simulink model "steercont_SAVIK_2019b_"  (R2020a)
settings: Solver=FixedStepAuto  StartTime=0.0  StopTime=270  FixedStep=stept  RelTol=1e-3
model workspace (MAT data in the model file):
  ip = Simulink.Signal
  ip.DataType = 'double'
  ip.Dimensions = [1 2]
  ip.DimensionsMode = 'auto'
  ip.Complexity = 'real'
  ip.SampleTime = -1
  ip.SamplingMode = 'auto'
values from neighbouring files (symbols this model uses):
  IC_theta0 = gamma_1+IC_theta1    (= 4.71238898038)    [purepursuit_waypoints.m]
  IC_theta1 = (3*pi)/2    (= 4.71238898038)    [purepursuit_waypoints.m]
  IC_x0 = IC_x0f-L_0f*cos(IC_theta0)    [purepursuit_waypoints.m]
  IC_x1 = 0    [purepursuit_waypoints.m]
  IC_y0 = IC_y0f-L_0f*sin(IC_theta0)    [purepursuit_waypoints.m]
  IC_y1 = 0    [purepursuit_waypoints.m]
  L_0b = 0.48    [purepursuit_waypoints.m]
  L_0f = 3.8    [purepursuit_waypoints.m]
  L_1f = 7.21    [purepursuit_waypoints.m]
  LD = 15    [purepursuit_waypoints.m]
  stept = 0.01    [purepursuit_waypoints.m]
  v_0 = -1    [purepursuit_waypoints.m]
  wayp = [0 0;0 20;20 20;20 -40; -40 -40; 0 -80]    [purepursuit_waypoints.m]
undefined symbols (not defined in the file or in its folder): DiscIntNeverNeededParam
settings Model: PauseTimes=0  OrderedModelArguments=off  Creator=giridhar  LastModifiedBy=giridhar
settings SolverCC: AlgebraicLoopSolver=LineSearch  MinimalZcImpactIntegration=on
settings DebuggingCC: ReadBeforeWriteMsg=DisableAll  WriteAfterWriteMsg=DisableAll  WriteAfterReadMsg=DisableAll  MultiTaskDSMMsg=none  SFUnusedDataAndEventsDiag=none
settings ModelReferenceCC: UpdateModelReferenceTargets=IfOutOfDate
settings SFSimCC: SFSimEcho=off

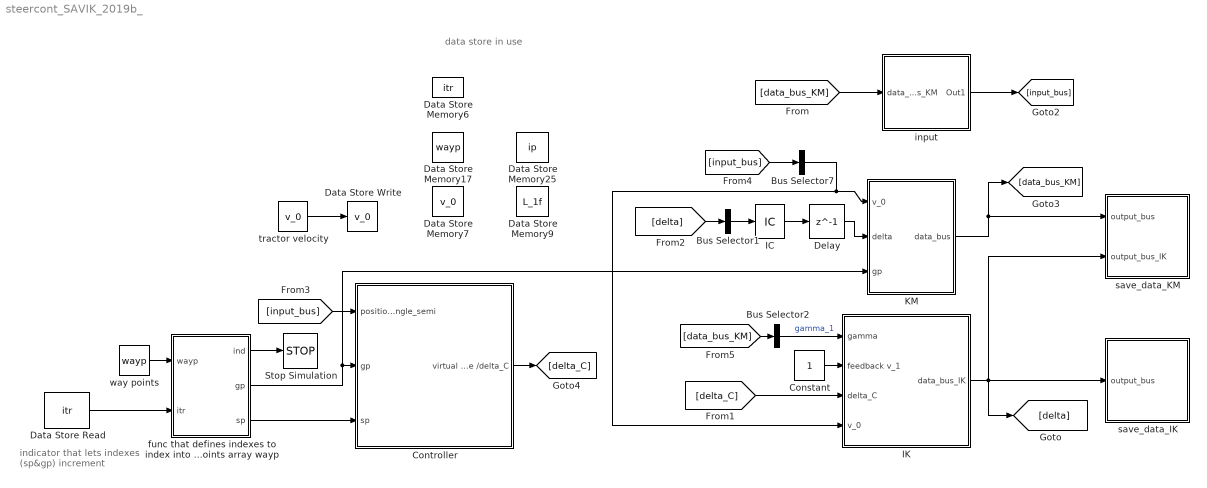
== system steercont_SAVIK_2019b_ ==
  note: indicator that lets indexes
      | (sp&gp) increment
  note: data store in use
  Bus Selector1 : BusSelector  OutputSignals=angle.steering_angle  OutputAsBus=on
  Bus Selector2 : BusSelector  OutputSignals=angle.articulation_angle  OutputAsBus=on
  Bus Selector7 : BusSelector  OutputSignals=u_0  OutputAsBus=on
  Constant : Constant
  Controller : Subsystem
  Data Store Memory17 : DataStoreMemory  DataStoreName=wayp  ReadBeforeWriteMsg=warning  WriteAfterWriteMsg=warning  WriteAfterReadMsg=warning  InitialValue=wayp  VectorParams1D=off  ShowAdditionalParam=off  OutDataTypeStr=double
  Data Store Memory25 : DataStoreMemory  DataStoreName=ip  ReadBeforeWriteMsg=warning  WriteAfterWriteMsg=warning  WriteAfterReadMsg=warning  InitialValue=[0 0]  VectorParams1D=off  ShowAdditionalParam=off  OutDataTypeStr=double  Dimensions=[1 2]  StateMustResolveToSignalObject=on
  Data Store Memory6 : DataStoreMemory  DataStoreName=itr  ReadBeforeWriteMsg=warning  WriteAfterWriteMsg=warning  WriteAfterReadMsg=warning  VectorParams1D=off  ShowAdditionalParam=off  OutDataTypeStr=double
  Data Store Memory7 : DataStoreMemory  DataStoreName=v_0  ReadBeforeWriteMsg=warning  WriteAfterWriteMsg=warning  WriteAfterReadMsg=warning  InitialValue=v_0  VectorParams1D=off  ShowAdditionalParam=off  OutDataTypeStr=double  Dimensions=[1 1]
  Data Store Memory9 : DataStoreMemory  DataStoreName=L_1f  ReadBeforeWriteMsg=warning  WriteAfterWriteMsg=warning  WriteAfterReadMsg=warning  InitialValue=7.21  VectorParams1D=off  ShowAdditionalParam=off  OutDataTypeStr=double  Dimensions=[1 1]
  Data Store Read : DataStoreRead  DataStoreName=itr
  Data Store Write : DataStoreWrite  DataStoreName=v_0
  Delay : Delay  DelayLength=1
  IC : InitialCondition  Value=0
  IK : Subsystem  SystemSampleTime=0.8
  KM : Subsystem  SystemSampleTime=0.8
  Stop Simulation : Stop
  func that defines indexes to index into waypoints array wayp : MATLAB Function
  input : Subsystem
  save_data_IK : Subsystem
  save_data_KM : Subsystem
  tractor velocity : Constant  Value=v_0
  way points : Constant  Value=wayp
  wires:
  [data_bus_KM] -> Bus Selector2/1
  input/1(Out1) -> [input_bus]
  KM/1(data_bus) -> [data_bus_KM], save_data_KM/1(output_bus)
  [delta] -> Bus Selector1/1
  IC/1 -> Delay/1
  Bus Selector2/1 -> IK/1(gamma)  "gamma_1"
  [input_bus] -> Controller/1(positions_yawangle_semi)
  Delay/1 -> KM/2(delta)
  Controller/1(virtual steer angle /delta_C) -> [delta_C]
  [input_bus] -> Bus Selector7/1
  [delta_C] -> IK/3(delta_C)
  [data_bus_KM] -> input/1(data_bus_KM)
  Bus Selector7/1 -> IK/4(v_0), KM/1(v_0)
  Bus Selector1/1 -> IC/1
  Constant/1 -> IK/2(feedback v_1)
  way points/1 -> func that defines indexes to index into waypoints array wayp/1(wayp)
  Data Store Read/1 -> func that defines indexes to index into waypoints array wayp/2(itr)
  func that defines indexes to index into waypoints array wayp/2(gp) -> Controller/2(gp), KM/3(gp)
  func that defines indexes to index into waypoints array wayp/3(sp) -> Controller/3(sp)
  func that defines indexes to index into waypoints array wayp/1(ind) -> Stop Simulation/1
  tractor velocity/1 -> Data Store Write/1
  IK/1(data_bus_IK) -> save_data_IK/1(output_bus), save_data_KM/2("output_bus_IK "), [delta]

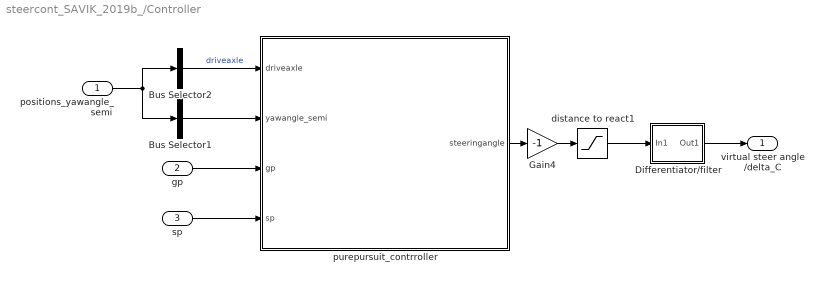
== system steercont_SAVIK_2019b_/Controller ==
  positions_yawangle_semi : Inport
  gp : Inport  Port=2
  sp : Inport  Port=3
  Bus Selector1 : BusSelector  OutputSignals=yawangle_semi  OutputAsBus=on
  Bus Selector2 : BusSelector  OutputSignals=positions  OutputAsBus=on
  Differentiator/filter : Subsystem  mask{ts=13.5}
      mask prompts: ts "response_time"
      mask init:
      | c=(3*pi/ts)^2;
  Gain4 : Gain  Gain=-1
  distance to react1 : Saturate  UpperLimit=1  LowerLimit=-1
  purepursuit_contrroller : Subsystem
  virtual steer angle /delta_C : Outport  PortDimensions=[1,1]  VectorParamsAs1DForOutWhenUnconnected=off
  wires:
  distance to react1/1 -> Differentiator/filter/1(In1)
  purepursuit_contrroller/1(steeringangle) -> Gain4/1
  Bus Selector2/1 -> purepursuit_contrroller/1(driveaxle)  "driveaxle"
  positions_yawangle_semi/1 -> Bus Selector1/1, Bus Selector2/1
  gp/1 -> purepursuit_contrroller/3(gp)
  sp/1 -> purepursuit_contrroller/4(sp)
  Gain4/1 -> distance to react1/1
  Bus Selector1/1 -> purepursuit_contrroller/2(yawangle_semi)
  Differentiator/filter/1(Out1) -> virtual steer angle /delta_C/1

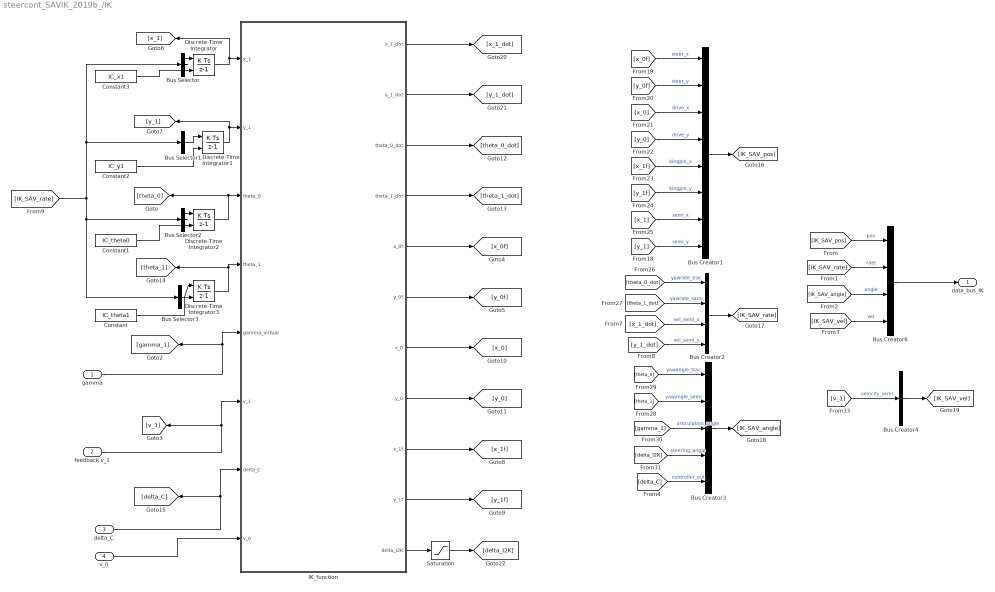
== system steercont_SAVIK_2019b_/IK ==
  gamma : Inport
  feedback v_1 : Inport  Port=2
  delta_C : Inport  Port=3
  v_0 : Inport  Port=4
  Bus Creator1 : BusCreator  Inputs=8
  Bus Creator2 : BusCreator  Inputs=4
  Bus Creator3 : BusCreator  Inputs=5
  Bus Creator4 : BusCreator  Inputs=1
  Bus Creator6 : BusCreator  Inputs=4
  Bus Selector : BusSelector  OutputSignals=vel_semi_x  OutputAsBus=on
  Bus Selector1 : BusSelector  OutputSignals=vel_semi_y  OutputAsBus=on
  Bus Selector2 : BusSelector  OutputSignals=yawrate_trac  OutputAsBus=on
  Bus Selector3 : BusSelector  OutputSignals=yawrate_semi  OutputAsBus=on
  Constant : Constant  Value=IC_theta1
  Constant1 : Constant  Value=IC_theta0
  Constant2 : Constant  Value=IC_y1
  Constant3 : Constant  Value=IC_x1
  Discrete-Time Integrator : DiscreteIntegrator  InitialConditionSource=external  InitialCondition=IC_x1  SampleTime=-1  ICPrevOutput=DiscIntNeverNeededParam  ICPrevScaledInput=DiscIntNeverNeededParam
  Discrete-Time Integrator1 : DiscreteIntegrator  InitialConditionSource=external  InitialCondition=IC_y1  SampleTime=-1  ICPrevOutput=DiscIntNeverNeededParam  ICPrevScaledInput=DiscIntNeverNeededParam
  Discrete-Time Integrator2 : DiscreteIntegrator  InitialConditionSource=external  InitialCondition=IC_theta0  SampleTime=-1  ICPrevOutput=DiscIntNeverNeededParam  ICPrevScaledInput=DiscIntNeverNeededParam
  Discrete-Time Integrator3 : DiscreteIntegrator  InitialConditionSource=external  InitialCondition=IC_theta1  SampleTime=-1  ICPrevOutput=DiscIntNeverNeededParam  ICPrevScaledInput=DiscIntNeverNeededParam
  IK_function : MATLAB Function  TreatAsAtomicUnit=on
  Saturation : Saturate  UpperLimit=0.7  LowerLimit=-0.7
  data_bus_IK : Outport  VectorParamsAs1DForOutWhenUnconnected=off
  wires:
  IK_function/7(x_0) -> [x_0]
  IK_function/8(y_0) -> [y_0]
  IK_function/1(x_1_dot) -> [x_1_dot]
  IK_function/10(y_1f) -> [y_1f]
  IK_function/9(x_1f) -> [x_1f]
  Discrete-Time Integrator/1 -> [x_1], IK_function/1(x_1)
  Discrete-Time Integrator1/1 -> [y_1], IK_function/2(y_1)
  gamma/1 -> [gamma_1], IK_function/5(gamma_virtual)
  IK_function/2(y_1_dot) -> [y_1_dot]
  delta_C/1 -> IK_function/7(delta_C), [delta_C]
  Discrete-Time Integrator3/1 -> IK_function/4(theta_1), [theta_1]
  IK_function/5(x_0f) -> [x_0f]
  IK_function/6(y_0f) -> [y_0f]
  [y_0f] -> Bus Creator1/2  "steer_y"
  [x_1f] -> Bus Creator1/5  "kingpin_x"
  Bus Creator6/1 -> data_bus_IK/1
  [v_1] -> Bus Creator4/1  "velocity_semi"
  [x_0] -> Bus Creator1/3  "drive_x"
  [y_1f] -> Bus Creator1/6  "kingpin_y"
  [x_0f] -> Bus Creator1/1  "steer_x"
  [y_0] -> Bus Creator1/4  "drive_y"
  Bus Creator3/1 -> [IK_SAV_angle]
  [theta_0_dot] -> Bus Creator2/1  "yawrate_trac"
  [theta_1_dot] -> Bus Creator2/2  "yawrate_semi"
  Discrete-Time Integrator2/1 -> [theta_0], IK_function/3(theta_0)
  [IK_SAV_rate] -> Bus Selector/1, Bus Selector1/1, Bus Selector3/1, Bus Selector2/1
  Bus Creator2/1 -> [IK_SAV_rate]
  Bus Creator1/1 -> [IK_SAV_pos]
  [delta_I2K] -> Bus Creator3/4  "steering_angle"
  [gamma_1] -> Bus Creator3/3  "articulation_angle"
  Bus Creator4/1 -> [IK_SAV_vel]
  [theta_1] -> Bus Creator3/2  "yawangle_semi"
  [IK_SAV_rate] -> Bus Creator6/2  "rate"
  [theta_0] -> Bus Creator3/1  "yawangle_trac"
  [IK_SAV_pos] -> Bus Creator6/1  "pos"
  [IK_SAV_angle] -> Bus Creator6/3  "angle"
  [IK_SAV_vel] -> Bus Creator6/4  "vel"
  Bus Selector3/1 -> Discrete-Time Integrator3/1
  Bus Selector2/1 -> Discrete-Time Integrator2/1
  Bus Selector/1 -> Discrete-Time Integrator/1
  Bus Selector1/1 -> Discrete-Time Integrator1/1
  [y_1_dot] -> Bus Creator2/4  "vel_semi_y"
  [x_1_dot] -> Bus Creator2/3  "vel_semi_x"
  IK_function/11(delta_I2K) -> Saturation/1
  [delta_C] -> Bus Creator3/5  "controller_out"
  feedback v_1/1 -> [v_1], IK_function/6(v_1)
  Saturation/1 -> [delta_I2K]
  [y_1] -> Bus Creator1/8  "semi_y"
  [x_1] -> Bus Creator1/7  "semi_x"
  Constant/1 -> Discrete-Time Integrator3/2
  Constant1/1 -> Discrete-Time Integrator2/2
  Constant2/1 -> Discrete-Time Integrator1/2
  Constant3/1 -> Discrete-Time Integrator/2
  v_0/1 -> IK_function/8(v_0)
  IK_function/4(theta_1_dot) -> [theta_1_dot]
  IK_function/3(theta_0_dot) -> [theta_0_dot]

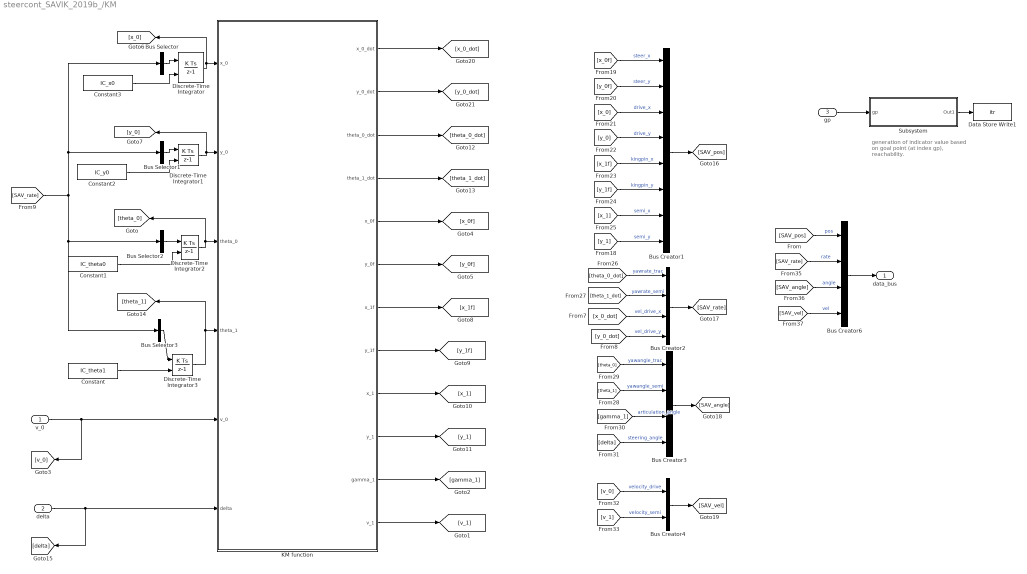
== system steercont_SAVIK_2019b_/KM ==
  note: generation of indicator value
      | based on goal point (at index gp),
      | reachability.
  v_0 : Inport
  delta : Inport  Port=2
  gp : Inport  Port=3
  Bus Creator1 : BusCreator  Inputs=8
  Bus Creator2 : BusCreator  Inputs=4
  Bus Creator3 : BusCreator  Inputs=4
  Bus Creator4 : BusCreator  Inputs=2
  Bus Creator6 : BusCreator  Inputs=4
  Bus Selector : BusSelector  OutputSignals=vel_drive_x  OutputAsBus=on
  Bus Selector1 : BusSelector  OutputSignals=vel_drive_y  OutputAsBus=on
  Bus Selector2 : BusSelector  OutputSignals=yawrate_trac  OutputAsBus=on
  Bus Selector3 : BusSelector  OutputSignals=yawrate_semi  OutputAsBus=on
  Constant : Constant  Value=IC_theta1
  Constant1 : Constant  Value=IC_theta0
  Constant2 : Constant  Value=IC_y0
  Constant3 : Constant  Value=IC_x0
  Data Store Write1 : DataStoreWrite  DataStoreName=itr
  Discrete-Time Integrator : DiscreteIntegrator  InitialConditionSource=external  InitialCondition=IC_x0  SampleTime=-1  ICPrevOutput=DiscIntNeverNeededParam  ICPrevScaledInput=DiscIntNeverNeededParam
  Discrete-Time Integrator1 : DiscreteIntegrator  InitialConditionSource=external  InitialCondition=IC_y0  SampleTime=-1  ICPrevOutput=DiscIntNeverNeededParam  ICPrevScaledInput=DiscIntNeverNeededParam
  Discrete-Time Integrator2 : DiscreteIntegrator  InitialConditionSource=external  InitialCondition=IC_theta0  SampleTime=-1  ICPrevOutput=DiscIntNeverNeededParam  ICPrevScaledInput=DiscIntNeverNeededParam
  Discrete-Time Integrator3 : DiscreteIntegrator  InitialConditionSource=external  InitialCondition=IC_theta1  SampleTime=-1  ICPrevOutput=DiscIntNeverNeededParam  ICPrevScaledInput=DiscIntNeverNeededParam
  KM function : MATLAB Function  TreatAsAtomicUnit=on
  Subsystem : Subsystem
  data_bus : Outport  VectorParamsAs1DForOutWhenUnconnected=off
  wires:
  KM function/9(x_1) -> [x_1]
  KM function/10(y_1) -> [y_1]
  KM function/1(x_0_dot) -> [x_0_dot]
  KM function/8(y_1f) -> [y_1f]
  KM function/7(x_1f) -> [x_1f]
  Discrete-Time Integrator/1 -> KM function/1(x_0), [x_0]
  Discrete-Time Integrator1/1 -> KM function/2(y_0), [y_0]
  KM function/11(gamma_1) -> [gamma_1]
  KM function/2(y_0_dot) -> [y_0_dot]
  delta/1 -> [delta], KM function/6(delta)
  Discrete-Time Integrator3/1 -> [theta_1], KM function/4(theta_1)
  KM function/5(x_0f) -> [x_0f]
  KM function/6(y_0f) -> [y_0f]
  v_0/1 -> [v_0], KM function/5(v_0)
  [y_0f] -> Bus Creator1/2  "steer_y"
  [x_1f] -> Bus Creator1/5  "kingpin_x"
  Bus Creator6/1 -> data_bus/1
  [v_1] -> Bus Creator4/2  "velocity_semi"
  [x_0] -> Bus Creator1/3  "drive_x"
  [y_1f] -> Bus Creator1/6  "kingpin_y"
  [x_0f] -> Bus Creator1/1  "steer_x"
  [y_0] -> Bus Creator1/4  "drive_y"
  Bus Creator3/1 -> [SAV_angle]
  [v_0] -> Bus Creator4/1  "velocity_drive"
  [theta_0_dot] -> Bus Creator2/1  "yawrate_trac"
  [theta_1_dot] -> Bus Creator2/2  "yawrate_semi"
  Discrete-Time Integrator2/1 -> [theta_0], KM function/3(theta_0)
  [SAV_rate] -> Bus Selector/1, Bus Selector1/1, Bus Selector3/1, Bus Selector2/1
  Bus Creator2/1 -> [SAV_rate]
  Bus Creator1/1 -> [SAV_pos]
  [delta] -> Bus Creator3/4  "steering_angle"
  [gamma_1] -> Bus Creator3/3  "articulation_angle"
  Bus Creator4/1 -> [SAV_vel]
  [theta_1] -> Bus Creator3/2  "yawangle_semi"
  [SAV_rate] -> Bus Creator6/2  "rate"
  [theta_0] -> Bus Creator3/1  "yawangle_trac"
  [SAV_pos] -> Bus Creator6/1  "pos"
  [SAV_angle] -> Bus Creator6/3  "angle"
  [SAV_vel] -> Bus Creator6/4  "vel"
  Bus Selector3/1 -> Discrete-Time Integrator3/1
  Bus Selector2/1 -> Discrete-Time Integrator2/1
  Bus Selector/1 -> Discrete-Time Integrator/1
  Bus Selector1/1 -> Discrete-Time Integrator1/1
  [y_0_dot] -> Bus Creator2/4  "vel_drive_y"
  [x_0_dot] -> Bus Creator2/3  "vel_drive_x"
  KM function/12(v_1) -> [v_1]
  [x_1] -> Bus Creator1/7  "semi_x"
  [y_1] -> Bus Creator1/8  "semi_y"
  Constant3/1 -> Discrete-Time Integrator/2
  Constant/1 -> Discrete-Time Integrator3/2
  Constant2/1 -> Discrete-Time Integrator1/2
  Constant1/1 -> Discrete-Time Integrator2/2
  Subsystem/1(Out1) -> Data Store Write1/1
  gp/1 -> Subsystem/1(gp)
  KM function/3(theta_0_dot) -> [theta_0_dot]
  KM function/4(theta_1_dot) -> [theta_1_dot]

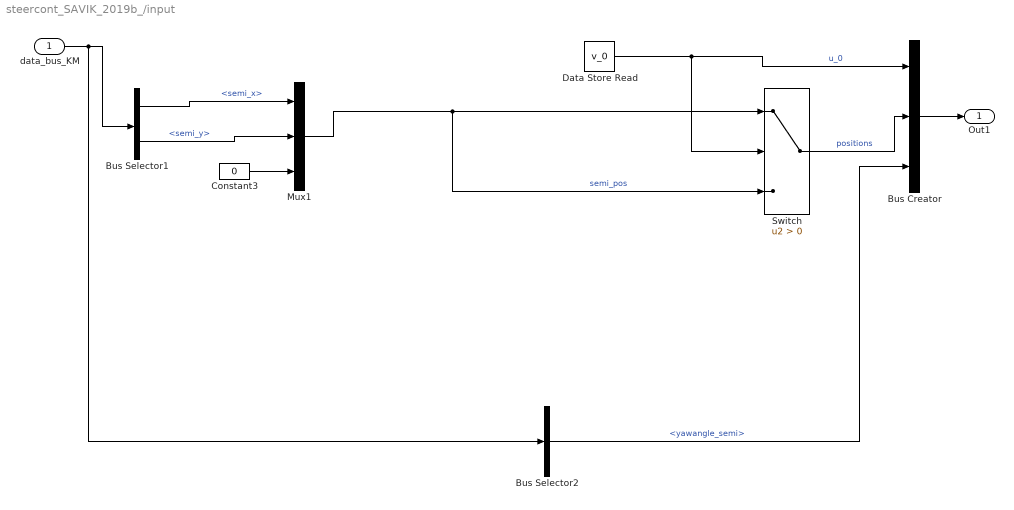
== system steercont_SAVIK_2019b_/input ==
  data_bus_KM : Inport
  Bus Creator : BusCreator  Inputs=3
  Bus Selector1 : BusSelector  OutputSignals=pos.semi_x,pos.semi_y
  Bus Selector2 : BusSelector  OutputSignals=angle.yawangle_semi
  Constant3 : Constant  Value=0
  Data Store Read : DataStoreRead  DataStoreName=v_0
  Mux1 : Mux  Inputs=3
  Switch : Switch  Criteria=u2 > Threshold
  Out1 : Outport  VectorParamsAs1DForOutWhenUnconnected=off
  wires:
  Data Store Read/1 -> Switch/2, Bus Creator/1  "u_0"
  Bus Creator/1 -> Out1/1
  Constant3/1 -> Mux1/3
  data_bus_KM/1 -> Bus Selector2/1, Bus Selector1/1
  Bus Selector1/1 -> Mux1/1  "<semi_x>"
  Bus Selector1/2 -> Mux1/2  "<semi_y>"
  Mux1/1 -> Switch/1, Switch/3  "semi_pos"
  Switch/1 -> Bus Creator/2  "positions"
  Bus Selector2/1 -> Bus Creator/3  "<yawangle_semi>"

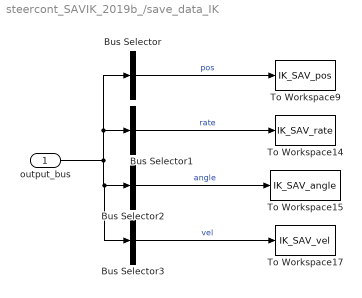
== system steercont_SAVIK_2019b_/save_data_IK ==
  output_bus : Inport
  Bus Selector : BusSelector  OutputSignals=pos.steer_x,pos.steer_y,pos.drive_x,pos.drive_y,pos.kingpin_x,pos.kingpin_y,pos.semi_x,pos.semi_y  OutputAsBus=on
  Bus Selector1 : BusSelector  OutputSignals=rate.yawrate_trac,rate.yawrate_semi,rate.vel_semi_x,rate.vel_semi_y  OutputAsBus=on
  Bus Selector2 : BusSelector  OutputSignals=angle.yawangle_trac,angle.yawangle_semi,angle.articulation_angle,angle.steering_angle,angle.controller_out  OutputAsBus=on
  Bus Selector3 : BusSelector  OutputSignals=vel.velocity_semi  OutputAsBus=on
  To Workspace14 : ToWorkspace  VariableName=IK_SAV_rate  SampleTime=-1
  To Workspace15 : ToWorkspace  VariableName=IK_SAV_angle  SampleTime=-1
  To Workspace17 : ToWorkspace  VariableName=IK_SAV_vel  SampleTime=-1
  To Workspace9 : ToWorkspace  VariableName=IK_SAV_pos  SampleTime=-1
  wires:
  Bus Selector3/1 -> To Workspace17/1  "vel"
  Bus Selector/1 -> To Workspace9/1  "pos"
  Bus Selector2/1 -> To Workspace15/1  "angle"
  Bus Selector1/1 -> To Workspace14/1  "rate"
  output_bus/1 -> Bus Selector/1, Bus Selector1/1, Bus Selector3/1, Bus Selector2/1

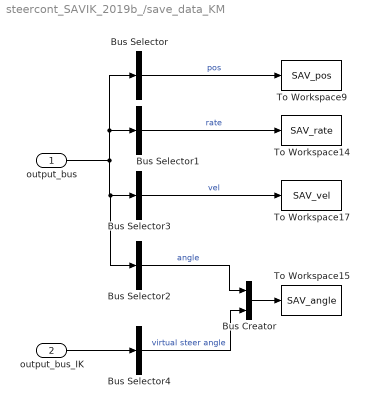
== system steercont_SAVIK_2019b_/save_data_KM ==
  output_bus : Inport
  "output_bus_IK " : Inport  Port=2
  Bus Creator : BusCreator  Inputs=2
  Bus Selector : BusSelector  OutputSignals=pos.steer_x,pos.steer_y,pos.drive_x,pos.drive_y,pos.kingpin_x,pos.kingpin_y,pos.semi_x,pos.semi_y  OutputAsBus=on
  Bus Selector1 : BusSelector  OutputSignals=rate.yawrate_trac,rate.yawrate_semi,rate.vel_drive_x,rate.vel_drive_y  OutputAsBus=on
  Bus Selector2 : BusSelector  OutputSignals=angle.yawangle_trac,angle.yawangle_semi,angle.articulation_angle,angle.steering_angle  OutputAsBus=on
  Bus Selector3 : BusSelector  OutputSignals=vel.velocity_drive,vel.velocity_semi  OutputAsBus=on
  Bus Selector4 : BusSelector  OutputSignals=angle.controller_out  OutputAsBus=on
  To Workspace14 : ToWorkspace  VariableName=SAV_rate  SampleTime=-1
  To Workspace15 : ToWorkspace  VariableName=SAV_angle  SampleTime=-1
  To Workspace17 : ToWorkspace  VariableName=SAV_vel  SampleTime=-1
  To Workspace9 : ToWorkspace  VariableName=SAV_pos  SampleTime=-1
  wires:
  output_bus/1 -> Bus Selector2/1, Bus Selector3/1, Bus Selector1/1, Bus Selector/1
  Bus Selector1/1 -> To Workspace14/1  "rate"
  Bus Selector/1 -> To Workspace9/1  "pos"
  Bus Selector3/1 -> To Workspace17/1  "vel"
  "output_bus_IK "/1 -> Bus Selector4/1
  Bus Creator/1 -> To Workspace15/1
  Bus Selector2/1 -> Bus Creator/1  "angle"
  Bus Selector4/1 -> Bus Creator/2  "virtual steer angle"

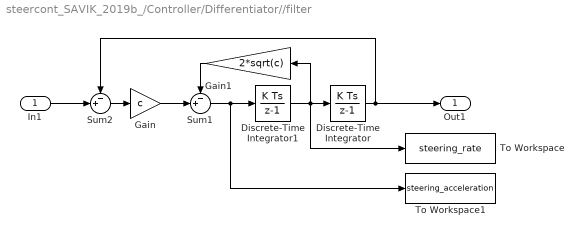
== system steercont_SAVIK_2019b_/Controller/Differentiator//filter ==
  In1 : Inport
  Discrete-Time Integrator : DiscreteIntegrator  SampleTime=-1  ICPrevOutput=DiscIntNeverNeededParam  ICPrevScaledInput=DiscIntNeverNeededParam
  Discrete-Time Integrator1 : DiscreteIntegrator  SampleTime=-1  ICPrevOutput=DiscIntNeverNeededParam  ICPrevScaledInput=DiscIntNeverNeededParam
  Gain : Gain  Gain=c  SaturateOnIntegerOverflow=on  OutDataTypeStr=Inherit: Same as input  ParamDataTypeStr=Inherit: Same as input
  Gain1 : Gain  Gain=2*sqrt(c)  SaturateOnIntegerOverflow=on  OutDataTypeStr=Inherit: Same as input  ParamDataTypeStr=Inherit: Same as input
  Sum1 : Sum  Inputs=-+|  SaturateOnIntegerOverflow=on
  Sum2 : Sum  Inputs=-+|  SaturateOnIntegerOverflow=on
  To Workspace : ToWorkspace  VariableName=steering_rate  SampleTime=-1
  To Workspace1 : ToWorkspace  VariableName=steering_acceleration  SampleTime=-1
  Out1 : Outport
  wires:
  Discrete-Time Integrator1/1 -> Discrete-Time Integrator/1, To Workspace/1, Gain1/1
  Discrete-Time Integrator/1 -> Out1/1, Sum2/1
  Sum1/1 -> Discrete-Time Integrator1/1, To Workspace1/1
  Sum2/1 -> Gain/1
  In1/1 -> Sum2/2
  Gain1/1 -> Sum1/1
  Gain/1 -> Sum1/2

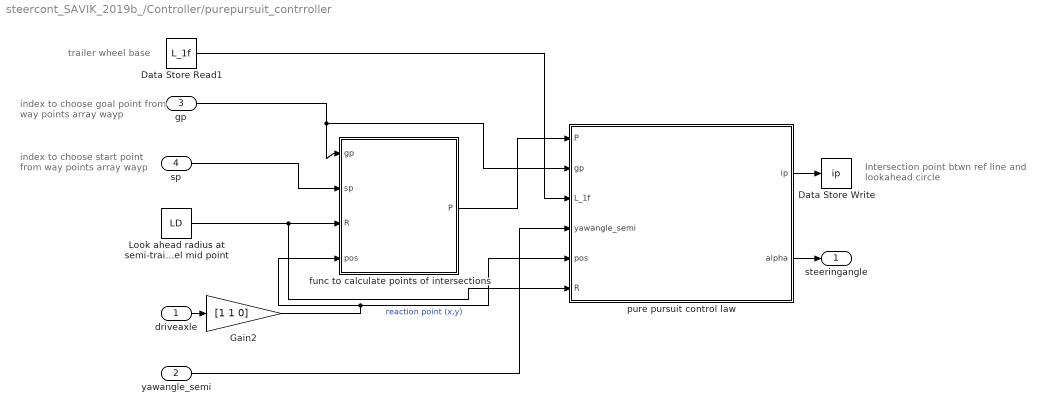
== system steercont_SAVIK_2019b_/Controller/purepursuit_contrroller ==
  note: index to choose goal point from
      | way points array wayp
  note: trailer wheel base
  note: Intersection point
      | btwn ref line and lookahead circle
  note: index to choose start point
      | from way points array wayp
  driveaxle : Inport
  yawangle_semi : Inport  Port=2
  gp : Inport  Port=3
  sp : Inport  Port=4
  Data Store Read1 : DataStoreRead  DataStoreName=L_1f
  Data Store Write : DataStoreWrite  DataStoreName=ip
  Gain2 : Gain  Gain=[1 1 0]
  Look ahead radius at semi-trailer axel mid point : Constant  Value=LD
  func to calculate points of intersections : MATLAB Function  TreatAsAtomicUnit=on
  pure pursuit control law : MATLAB Function  TreatAsAtomicUnit=on
  steeringangle : Outport  VectorParamsAs1DForOutWhenUnconnected=off
  wires:
  Data Store Read1/1 -> pure pursuit control law/3(L_1f)
  func to calculate points of intersections/1(P) -> pure pursuit control law/1(P)
  pure pursuit control law/1(ip) -> Data Store Write/1
  Look ahead radius at semi-trailer axel mid point/1 -> func to calculate points of intersections/3(R), pure pursuit control law/6(R)
  pure pursuit control law/2(alpha) -> steeringangle/1
  gp/1 -> func to calculate points of intersections/1(gp), pure pursuit control law/2(gp)
  Gain2/1 -> func to calculate points of intersections/4(pos), pure pursuit control law/5(pos)  "reaction point (x,y)"
  driveaxle/1 -> Gain2/1
  yawangle_semi/1 -> pure pursuit control law/4(yawangle_semi)
  sp/1 -> func to calculate points of intersections/2(sp)

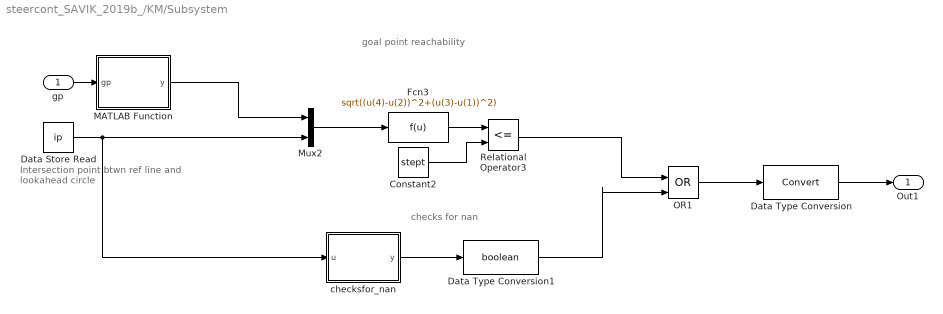
== system steercont_SAVIK_2019b_/KM/Subsystem ==
  note: Intersection point
      | btwn ref line and lookahead circle
  note: checks for nan
  note: goal point reachability
  gp : Inport
  Constant2 : Constant  Value=stept
  Data Store Read : DataStoreRead  DataStoreName=ip
  Data Type Conversion : DataTypeConversion
  Data Type Conversion1 : DataTypeConversion  OutDataTypeStr=boolean
  Fcn3 : Fcn  Expr=sqrt((u(4)-u(2))^2+(u(3)-u(1))^2)
  MATLAB Function : MATLAB Function  TreatAsAtomicUnit=on
  Mux2 : Mux  Inputs=2
  OR1 : Logic  Operator=OR  IconShape=distinctive  AllPortsSameDT=off  OutDataTypeStr=boolean
  Relational Operator3 : RelationalOperator  Operator=<=  OutDataTypeStr=boolean  RndMeth=Simplest
  checksfor_nan : MATLAB Function  TreatAsAtomicUnit=on
  Out1 : Outport
  wires:
  OR1/1 -> Data Type Conversion/1
  Data Type Conversion/1 -> Out1/1
  Data Store Read/1 -> checksfor_nan/1(u), Mux2/2
  Fcn3/1 -> Relational Operator3/1
  gp/1 -> MATLAB Function/1(gp)
  Constant2/1 -> Relational Operator3/2
  Mux2/1 -> Fcn3/1
  Relational Operator3/1 -> OR1/1
  checksfor_nan/1(y) -> Data Type Conversion1/1
  Data Type Conversion1/1 -> OR1/2
  MATLAB Function/1(y) -> Mux2/1

== matlab function steercont_SAVIK_2019b_/KM/KM function ==
  data: x_0 input; y_0 input; theta_0 input; theta_1 input; x_0_dot output; L_0b parameter; L_1f parameter; y_0_dot output; theta_0_dot output; theta_1_dot output; v_0 input; x_0f output; y_0f output; x_1f output; y_1f output; x_1 output; y_1 output; gamma_1 output; v_1 output; delta input; L_0f parameter
% The vehicle is described in global coordinates for which ISO system is used.
% Yaw rates can be derived from applying non-holonomic consraint (no lateral
% slip) on each axle.

function [x_0_dot,y_0_dot,theta_0_dot,theta_1_dot,x_0f,y_0f,x_1f,y_1f,x_1,y_1,gamma_1,...
         v_1] = vehicle(x_0,y_0,theta_0,theta_1,L_0b, L_1f, v_0,delta, L_0f)
     
%_______________________ position _________________________________________
% steer axle

        x_0f = x_0+L_0f*cos(theta_0);
        y_0f = y_0+L_0f*sin(theta_0);
        
%king-pin

        x_1f = x_0+L_0b*cos(theta_0);
        y_1f = y_0+L_0b*sin(theta_0);
 
% semitrailer axle

        x_1 = x_1f-L_1f*cos(theta_1);
        y_1 = y_1f-L_1f*sin(theta_1);
        
% articulation angle
        
        gamma_1 = (theta_0-theta_1);                                        % articulation angle
        
% yaw rate        
        
        theta_0_dot = (v_0/L_0f) * tan(delta);                              % tractor 
        theta_1_dot = (v_0/L_1f)*sin(gamma_1) + (L_0b/L_1f)*...
                        (theta_0_dot)*cos(gamma_1);                         % semitrailer                            
                    
                    
% semitrailer longitudinal velocity in its own local body coordinate system

        v_1 = v_0;  
                    
        
%_________________________next iteration____________________________________
        
        x_0_dot = v_0 * cos(theta_0);                                          % tractor drive axle velocity in global x-direction
        y_0_dot = v_0 * sin(theta_0);                                          % tractor drive axle velocity in global y-direction

== matlab function steercont_SAVIK_2019b_/KM/Subsystem/checksfor_nan ==
  data: u input; y output
function y = fcn(u)
if any(isnan(u), 'all')
    y=1;
else
    y=0;
end

== matlab function steercont_SAVIK_2019b_/func that defines indexes to index into waypoints array wayp ==
  data: ind output; wayp input; gp output; itr input; sp output
function [ind,gp,sp] = fcn(wayp,itr)

ind=0;           %stops simulation when ind=1;
%defining index values sp for start point and gp for goal point,that index
%into wayp later on
persistent j
if isempty(j)
    j=1;
end
if itr==1
j = j+1;
end
i=j;

szwayp=size(wayp,1);
sp=i;


if i<szwayp
ind=0;
gp=i+1;
else
    ind=1;        %stops simulation when ind=1;
    gp=i-1;
end

== matlab function steercont_SAVIK_2019b_/KM/Subsystem/MATLAB Function ==
  data: gp input; y output; wayp data_store_memory
function y = fcn(gp)
global wayp
y=wayp(gp,:);

== matlab function steercont_SAVIK_2019b_/Controller/purepursuit_contrroller/func to calculate points of intersections ==
  data: gp input; sp input; R input; P output; pos input; wayp data_store_memory
function P = calc_ips(gp, sp, R,pos)
%this func calculates points of intersection between ref line (formed
%with goal point, start point) and look ahead circle with center at semitrailer axel midpoint  
global wayp
P=zeros(2,2);
%indexing into wayp with indexes gp and sp
p1=[wayp(gp,1) wayp(gp,2)];
p2=[wayp(sp,1) wayp(sp,2)];
slope = (p1(1,2)-p2(1,2))/(p1(1,1)-p2(1,1));
if slope == -inf || slope ==inf
    intercpt=p1(1,1);
else
intercpt = p2(1,2)-slope*p2(1,1);
end
%updating center of circle with the current pose of semitrailer axle
%position
centerx=pos(1,1);
centery=pos(2,1);
radius=R;
%linecirc is a function that caluculates point of intersection between line
%and circle, line is defined with 
coder.extrinsic('linecirc')
[xout,yout] = linecirc(slope,intercpt,centerx,centery,radius);
P=[xout ; yout];

== matlab function steercont_SAVIK_2019b_/Controller/purepursuit_contrroller/pure pursuit control law ==
  data: ip output; P input size=[2 2]; alpha output size=[1,1]; gp input size=[1 1]; L_1f input; yawangle_semi input; pos input; R input; wayp data_store_memory
function [ip,alpha] = controlleroutput(P,gp,L_1f,yawangle_semi,pos,R)
%this func calculates steer angle that pursues the ref line formed between
%start point and goal point chosen from wayp
global wayp
Psz=size(P,2);          %num of intersection points, with x_cords in 1st column y_cords in 2nd column in matrix P
gp_cords=wayp(gp,:);
%now we need to find one point of intersection from the available two point
%of intersections. we choose the point of intersection that is close to the
%current goal point gp_cords with index number gp
distarray=zeros(Psz,3); % intersection points distance to gp (goal point)
 for k=1:Psz
     distarray(k,1:2)=[P(1,k) P(2,k)];
     distarray(k,3)=sqrt((P(1,k)-gp_cords(1,1))^2+(P(2,k)-gp_cords(1,2))^2);
 end
%choosing the nearest intersection point to the goal point from the
%available 2 points of intersection between reference line and look ahead
%circle
sortP=sortrows(distarray,3);  
ip=sortP(1,1:2);
alpha=zeros(1,1);
%Theta_e
num=ip(1,1)-pos(1,1);
den=ip(1,2)-pos(2,1);
theta_e = atan2(den,num)-yawangle_semi;   %orientation error
%simple pure pursuit control law 
alpha = -atan((2*L_1f*sin(theta_e))/R);   %steer angle that aims to reduce orientation error

== matlab function steercont_SAVIK_2019b_/IK/IK_function ==
  data: x_1 input; y_1 input; theta_0 input; theta_1 input; x_1_dot output; gamma_virtual input; y_1_dot output; theta_0_dot output; theta_1_dot output; v_1 input; x_0f output; y_0f output; x_0 output; y_0 output; x_1f output; y_1f output; delta_C input; delta_I2K output; v_0 input
% The vehicle is described in global coordinates for which ISO system is used.
% Yaw rates can be derived from applying non-holonomic consraint (no lateral
% slip) on each axle.

function [x_1_dot,y_1_dot,theta_0_dot,theta_1_dot,x_0f,y_0f,x_0,y_0,x_1f,y_1f,...
         delta_I2K] = vehicle(x_1,y_1,theta_0,theta_1,gamma_virtual,v_1,delta_C, v_0)
     
L_0f = 3.8;  %(tractor wheelbase)
L_1f = 7.21; %(trailer wheel base)
L_0b = 0.48;
     %_______________________ position _________________________________________
%king-pin

        x_1f = x_1+L_1f*cos(theta_1);
        y_1f = y_1+L_1f*sin(theta_1);

 
% drive axle

        x_0 = x_1f-L_0b*cos(theta_0);
        y_0 = y_1f-L_0b*sin(theta_0);

% steer axle

        x_0f = x_0+L_0f*cos(theta_0);
        y_0f = y_0+L_0f*sin(theta_0);
                       
% yaw rate        
                                      
        theta_1_dot = abs(v_1)*tan(delta_C)/L_1f;                           % semitrailer
        theta_0_dot = sign(v_1)*sign(L_0b)*(-(v_1/L_0b)*sin(gamma_virtual)+...
                    (L_1f/L_0b)*(theta_1_dot)*cos(gamma_virtual));                % tractor 
                     
% semitrailer longitudinal velocity in its own local body coordinate system

       
        
        delta_I2K = atan(L_0f*theta_0_dot/v_0);
                    
        
%_________________________next iteration___________________________________
        
        x_1_dot = v_1 * cos(theta_1);                                       % tractor drive axle velocity in global x-direction
        y_1_dot = v_1 * sin(theta_1);                                       % tractor drive axle velocity in global y-direction
